simulink library "ETF_Library"  (R2025a)
settings: Solver=VariableStepAuto  StartTime=0.0  StopTime=10.0  RelTol=1e-3
settings Model: Creator=damerius  LastModifiedBy=damerius
settings SFSimCC: SimTargetLang=C++  SimDLTargetLibrary=mkl-dnn

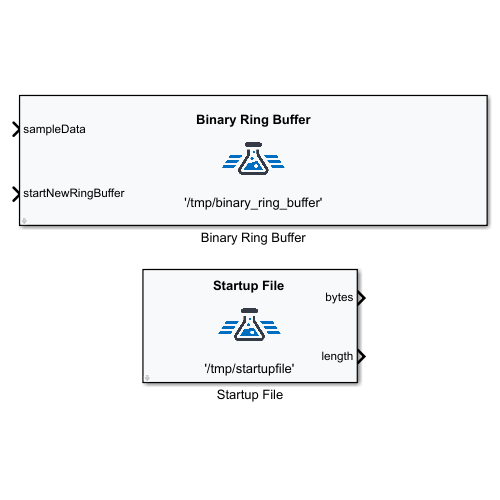
[thumbnail: Simulink's stored preview of the top-level diagram]
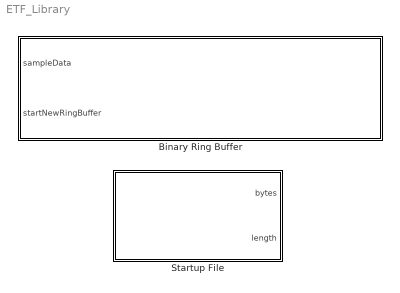
== system ETF_Library ==
  Binary Ring Buffer : Subsystem  mask{folderName='/tmp/binary_ring_buffer', threadPriority=20, sampleSize=1, numSamplesPerFile=1, numFiles=1, showDetails=off}
      mask prompts: folderName "Storage location:"; threadPriority "Worker thread priority (1 (lowest) ... 99 (highest), default is 20):"; sampleSize "Bytes per sample:"; numSamplesPerFile "Samples per file:"; numFiles "Files per ring buffer:"; showDetails "Show details output port"
      mask help:
      | Ring buffer for storing binary data samples in a non-blocking manner. All incoming samples are stored in memory and written to disk by a worker thread. The ring buffer can be re-initialized at any time to start a new ring buffer. All data files are stored in a specified folder, with each ring buffer instance creating a new subfolder named according to the current UTC time.<br><br>
      |
      | <b>sampleData</b><br>
      | Vector of bytes (uint8) that represent one data sample to be stored to the ring buffer. The dimension must be equal to the bytes-per-sample specified by this mask.<br><br>
      |
      | <b>startNewRingBuffer</b><br>
      | True if a new ring buffer should be started before writing the data sample. A new ring buffer is stored in a new subdirectory.<br><br>
      |
      | <b>details.isOpen</b><br>
      | True if the ring buffer is open, e.g. all files have been created successfully.<br><br>
      |
      | <b>details.numCachedSamples</b><br>
      | Number of cached samples in RAM that are waiting for to be written to the disk by the worker thread.
      mask init:
      | outPortDetails = find_system(gcb, 'LookUnderMasks','on','FollowLinks','on','Name','details');
      |     termPortDetails = find_system(gcb, 'LookUnderMasks','on','FollowLinks','on','Name','Terminator');
      |     hOut = get_param([gcb,'/BusCreator'],'PortHandles');
      |     if(showDetails)
      |         if(~isempty(termPortDetails))
      |             hIn = get_param([gcb,'/Terminator'],'PortHandles');
      |             delete_line(gcb,hOut.Outport(1),hIn.Inport(1));
      |             delete_block(termPortDetails);
      |         end
      |         if(isempty(outPortDetails))
      |             add_block('built-in/Outport',[gcb,'/details']);
      |             hIn = get_param([gcb,'/details'],'PortHandles');
      |             add_line(gcb,hOut.Outport(1),hIn.Inport(1));
      |             set_param([gcb,'/details'],'Port','1');
      |             set_param([gcb,'/details'],'Position',[10 33 40 47]);
      |         end
      |     else
      |         if(~isempty(outPortDetails))
      |             hIn = get_param([gcb,'/details'],'PortHandles');
      |             delete_line(gcb,hOut.Outport(1),hIn.Inport(1));
      |             delete_block(outPortDetails);
      |         end
      |         if(isempty(termPortDetails))
      |             add_block('built-in/Terminator',[gcb,'/Terminator']);
      |             hIn = get_param([gcb,'/Terminator'],'PortHandles');
      |             add_line(gcb,hOut.Outport(1),hIn.Inport(1));
      |             set_param([gcb,'/Terminator'],'Position',[15 30 35 50]);
      |         end
      |     end
      mask DialogControl DescGroupVar Prompt: Binary Ring Buffer
      mask DialogControl Container4 Prompt: Optional output
      mask DialogControl showDetails Tooltip: Check to enable the details output port.
      mask DialogControl folderName Tooltip: Path where to store the ring buffer files.
      mask DialogControl threadPriority Tooltip: Priority of the worker thread that writes cached sample data to the disk.
      mask DialogControl Container3 Prompt: Ring buffer size
      mask DialogControl sampleSize Tooltip: The number of bytes that represent one data sample.
      mask DialogControl numSamplesPerFile Tooltip: The total number of samples that are stored in one file.
      mask DialogControl numFiles Tooltip: The total number of files the ring buffer should contain.
      mask Display:
      | % Get dimension of block
      | pos = get_param(gcb, 'Position');
      | width = pos(3) - pos(1);
      | height = pos(4) - pos(2);
      | 
      | % Set image to center of block
      | imgSize = 48;
      | image('ETF_Icon.svg', [0.5*(width-imgSize),0.5*(height-imgSize),imgSize,imgSize]);
      | 
      | % Block title
      | text(0.5*width,0.5*(height+imgSize)+2, '{\bfBinary Ring Buffer}','horizontalAlignment','center','verticalAlignment','bottom','texmode','on');
      | 
      | % Show storage location
      | strText = get_param(gcb,'folderName');
      | text(0.5*width,0.5*(height-imgSize)-2,strText, 'horizontalAlignment','center','verticalAlignment','top');
  Startup File : Subsystem  mask{fileName='/tmp/startupfile', maxNumBytes=32}
      mask prompts: fileName "Filename (absolute path):"; maxNumBytes "Maximum number of bytes to read:"
      mask help:
      | This block reads a file in binary mode at startup, e.g. during the initialization step of the model. The binary data is stored in a buffer. During execution the buffer is available at the output ports.<br><br>
      | <b>bytes</b><br>
      | The array containing the binary content of the file.<br><br>
      | <b>length</b><br>
      | Actual number of bytes in the output array that represent the binary data.
      mask DialogControl DescGroupVar Prompt: Startup File
      mask DialogControl fileName Tooltip: Absolute path to the startup file.
      mask Display:
      | % Get dimension of block
      | pos = get_param(gcb, 'Position');
      | width = pos(3) - pos(1);
      | height = pos(4) - pos(2);
      | 
      | % Set image to center of block
      | imgSize = 48;
      | image('ETF_Icon.svg', [0.5*(width-imgSize),0.5*(height-imgSize),imgSize,imgSize]);
      | 
      | % Block title
      | text(0.5*width,0.5*(height+imgSize)+2, '{\bfStartup File}','horizontalAlignment','center','verticalAlignment','bottom','texmode','on');
      | 
      | % Show storage location
      | strText = get_param(gcb,'fileName');
      | text(0.5*width,0.5*(height-imgSize)-2,strText, 'horizontalAlignment','center','verticalAlignment','top');

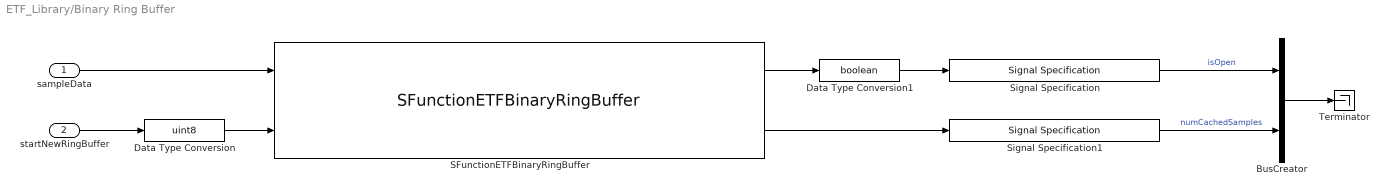
== system ETF_Library/Binary Ring Buffer ==
  sampleData : Inport  OutDataTypeStr=uint8  PortDimensions=sampleSize
  startNewRingBuffer : Inport  Port=2  OutDataTypeStr=boolean  PortDimensions=1
  BusCreator : BusCreator  Inputs=2
  Data Type Conversion : DataTypeConversion  OutDataTypeStr=uint8  SaturateOnIntegerOverflow=off  RndMeth=Floor
  Data Type Conversion1 : DataTypeConversion  OutDataTypeStr=boolean  SaturateOnIntegerOverflow=off  RndMeth=Floor
  SFunctionETFBinaryRingBuffer : S-Function  FunctionName=SFunctionETFBinaryRingBuffer  Parameters=SParameter1, SParameter2, SParameter3, SParameter4, SParameter5, SParameter6  SFunctionDeploymentMode=off  EnableBusSupport=off  mask(Legacy Function){SFunctionSpec=void ETFDriver_BinaryRingBufferStep(void* work1, uint8 y1[1], uint32 y2[1], uint8 u1[], uint8 u2), SParameter1=uint8(folderName), SParameter2=uint32(numel(folderName)), SParameter3=uint32(sampleSize), SParameter4=uint32(numSamplesPerFile), SParameter5=uint32(numFiles), SParameter6=int32(threadPriority), ShowSpec=on}
      mask prompts: SParameter1 "P1:"; SParameter2 "P2:"; SParameter3 "P3:"; SParameter4 "P4:"; SParameter5 "P5:"; SParameter6 "P6:"; ShowSpec "Display function specification"
      mask help:
      | This block allows you to call the legacy functions specified by the following Legacy Code Tool definition:
      | def.SFunctionName = 'SFunctionETFBinaryRingBuffer';
      | def.OutputFcnSpec = 'void ETFDriver_BinaryRingBufferStep(void* work1, uint8 y1[1], uint32 y2[1], uint8 u1[], uint8 u2)';
      | def.StartFcnSpec = 'void ETFDriver_BinaryRingBufferInitialize(void** work1, uint8 p1[], uint32 p2, uint32 p3, uint32 p4, uint32 p5, int32 p6)';
      | def.TerminateFcnSpec = 'void ETFDriver_BinaryRingBufferTerminate(void* work1)';
      | def.HeaderFiles = {'ETFDriver_BinaryRingBuffer.hpp'};
      | def.SourceFiles = {'ETFDriver_BinaryRingBuffer.cpp'};
      | def.IncPaths = {'etf'};
      | def.SrcPaths = {'etf'};
      | def.Options.useTlcWithAccel = false;
      mask Help: <p>This block was generated automatically by the Legacy Code Tool. For detailed help on this tool, call<a href="matlab:legacy_code('help')"> legacy_code('help')</a>.</p>
      mask Callback ShowSpec:
      | if strcmp(get_param(gcbh, 'ShowSpec'), 'on')
      |   set_param(gcbh, 'MaskDisplay', sprintf('fprintf(''%s'');', get_param(gcbh, 'SFunctionSpec')));
      | else
      |   set_param(gcbh, 'MaskDisplay', sprintf('fprintf(''%s'');', get_param(gcbh, 'FunctionName')));
      | end
      mask Display: fprintf('void ETFDriver_BinaryRingBufferStep(void* work1, uint8 y1[1], uint32 y2[1], uint8 u1[], uint8 u2)');
  Signal Specification : SignalSpecification  OutDataTypeStr=boolean  Dimensions=1
  Signal Specification1 : SignalSpecification  OutDataTypeStr=uint32  Dimensions=1
  Terminator : Terminator
  wires:
  Signal Specification1/1 -> BusCreator/2  "numCachedSamples"
  startNewRingBuffer/1 -> Data Type Conversion/1
  sampleData/1 -> SFunctionETFBinaryRingBuffer/1
  Data Type Conversion/1 -> SFunctionETFBinaryRingBuffer/2
  SFunctionETFBinaryRingBuffer/1 -> Data Type Conversion1/1
  Signal Specification/1 -> BusCreator/1  "isOpen"
  BusCreator/1 -> Terminator/1
  Data Type Conversion1/1 -> Signal Specification/1
  SFunctionETFBinaryRingBuffer/2 -> Signal Specification1/1

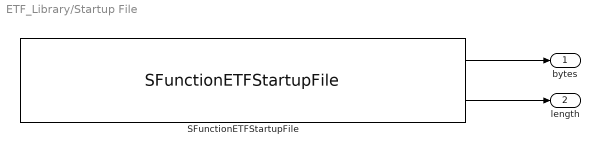
== system ETF_Library/Startup File ==
  SFunctionETFStartupFile : S-Function  FunctionName=SFunctionETFStartupFile  Parameters=SParameter1, SParameter2, SParameter3  SFunctionDeploymentMode=off  EnableBusSupport=off  mask(Legacy Function){SFunctionSpec=void ETFDriver_StartupFileStep(void* work1, uint8 y1[p3], uint32 y2[1], uint32 p3), SParameter1=uint8(fileName), SParameter2=uint32(numel(fileName)), SParameter3=uint32(maxNumBytes), ShowSpec=on}
      mask prompts: SParameter1 "P1:"; SParameter2 "P2:"; SParameter3 "P3:"; ShowSpec "Display function specification"
      mask help:
      | This block allows you to call the legacy functions specified by the following Legacy Code Tool definition:
      | def.SFunctionName = 'SFunctionETFStartupFile';
      | def.OutputFcnSpec = 'void ETFDriver_StartupFileStep(void* work1, uint8 y1[p3], uint32 y2[1], uint32 p3)';
      | def.StartFcnSpec = 'void ETFDriver_StartupFileInitialize(void** work1, uint8 p1[], uint32 p2, uint32 p3)';
      | def.TerminateFcnSpec = 'void ETFDriver_StartupFileTerminate(void* work1)';
      | def.HeaderFiles = {'ETFDriver_StartupFile.hpp'};
      | def.SourceFiles = {'ETFDriver_StartupFile.cpp'};
      | def.IncPaths = {'etf'};
      | def.SrcPaths = {'etf'};
      | def.Options.useTlcWithAccel = false;
      mask Help: <p>This block was generated automatically by the Legacy Code Tool. For detailed help on this tool, call<a href="matlab:legacy_code('help')"> legacy_code('help')</a>.</p>
      mask Callback ShowSpec:
      | if strcmp(get_param(gcbh, 'ShowSpec'), 'on')
      |   set_param(gcbh, 'MaskDisplay', sprintf('fprintf(''%s'');', get_param(gcbh, 'SFunctionSpec')));
      | else
      |   set_param(gcbh, 'MaskDisplay', sprintf('fprintf(''%s'');', get_param(gcbh, 'FunctionName')));
      | end
      mask Display: fprintf('void ETFDriver_StartupFileStep(void* work1, uint8 y1[p3], uint32 y2[1], uint32 p3)');
  bytes : Outport  OutDataTypeStr=uint8  PortDimensions=maxNumBytes
  length : Outport  Port=2  OutDataTypeStr=uint32  PortDimensions=1
  wires:
  SFunctionETFStartupFile/1 -> bytes/1
  SFunctionETFStartupFile/2 -> length/1
